simulink model "sistema"  (R2022b)
settings: Solver=ode4  StartTime=0.0  StopTime=4  FixedStep=1e-2  RelTol=1e-3  EnableMultiTasking=on
undefined symbols (not defined in the file): a, B, ft, K, l0, Lprime, M, R
settings Model: Creator=11802972  LastModifiedBy=andre
settings SolverCC: AlgebraicLoopSolver=TrustRegion
settings DataIOCC: LimitDataPoints=on  SaveFormat=Array  ReturnWorkspaceOutputs=off
settings OptimizationCC: LifeSpan=inf
settings DebuggingCC: UnconnectedInputMsg=warning  UnconnectedOutputMsg=warning  UnconnectedLineMsg=warning  SFUnexpectedBacktrackingDiag=warning  SFNoUnconditionalDefaultTransitionDiag=warning  SFExecutionAtInitializationDiag=none  SFMachineParentedDataDiag=warning  ArithmeticOperatorsInVariantConditions=warning
settings HardwareCC: ProdBitPerPointer=32  ProdBitPerSizeT=32  ProdBitPerPtrDiffT=32  ProdLargestAtomicFloat=None  ProdIntDivRoundTo=Undefined  ProdEndianess=Unspecified  ProdWordSize=32  ProdHWDeviceType=32-bit Generic
settings ModelReferenceCC: PropagateSignalLabelsOutOfModel=off
settings SFSimCC: SimUseLocalCustomCode=off  CustomCodeUndefinedFunction=UseInterfaceOnly
settings RTWCC: RTWUseLocalCustomCode=off
settings CodeAppCC: StateflowObjectComments=on
settings GRTTargetCC: TargetLangStandard=C89/C90 (ANSI)
settings ConfigComp: CovMetricSettings=dw  CovSaveCumulativeToWorkspaceVar=on  CovSaveSingleToWorkspaceVar=on  CovExternalEMLEnable=off

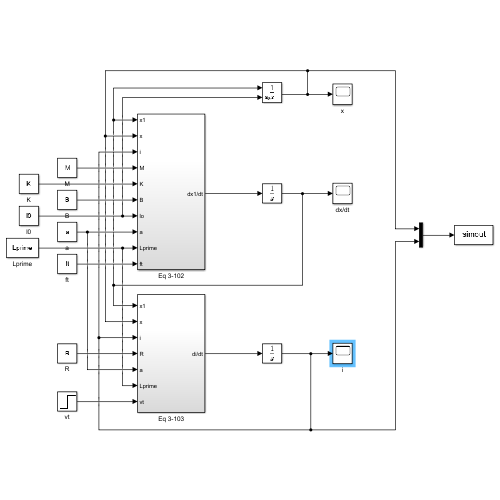
[thumbnail: Simulink's stored preview of the top-level diagram]
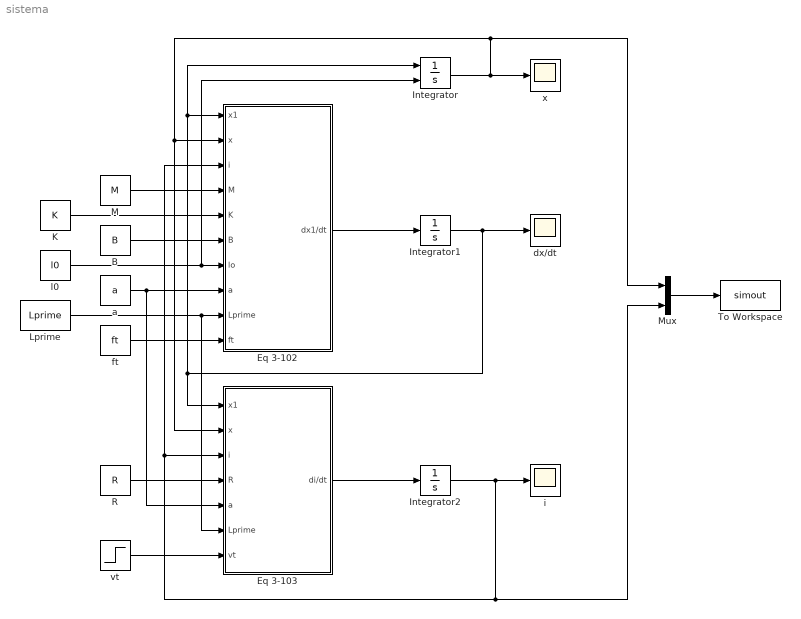
== system sistema ==
  B : Constant  Value=B
  "Eq 3-102 " : Subsystem
  Eq 3-103 : Subsystem
  Integrator : Integrator  InitialConditionSource=external
  Integrator1 : Integrator
  Integrator2 : Integrator
  K : Constant  Value=K
  Lprime : Constant  Value=Lprime
  M : Constant  Value=M
  Mux : Mux  Inputs=2
  R : Constant  Value=R
  To Workspace : ToWorkspace  VariableName=simout  SaveFormat=Timeseries  SampleTime=-1
  a : Constant  Value=a
  dx/dt : Scope
  ft : Constant  Value=ft
  i : Scope
  l0 : Constant  Value=l0
  "vt " : Step  Time=0.5  After=10  SampleTime=0
  x : Scope
  wires:
  M/1 -> "Eq 3-102 "/4(M)
  K/1 -> "Eq 3-102 "/5(K)
  B/1 -> "Eq 3-102 "/6(B)
  l0/1 -> Integrator/2, "Eq 3-102 "/7(lo)
  a/1 -> Eq 3-103/5(a), "Eq 3-102 "/8(a)
  ft/1 -> "Eq 3-102 "/10(ft)
  Lprime/1 -> Eq 3-103/6(Lprime), "Eq 3-102 "/9(Lprime)
  R/1 -> Eq 3-103/4(R)
  "vt "/1 -> Eq 3-103/7(vt)
  Integrator/1 -> Eq 3-103/2(x), "Eq 3-102 "/2(x), Mux/1, x/1
  "Eq 3-102 "/1(dx1/dt) -> Integrator1/1
  Integrator1/1 -> Eq 3-103/1(x1), Integrator/1, "Eq 3-102 "/1(x1), dx/dt/1
  Eq 3-103/1(di/dt) -> Integrator2/1
  Integrator2/1 -> Eq 3-103/3(i), "Eq 3-102 "/3(i), Mux/2, i/1
  Mux/1 -> To Workspace/1

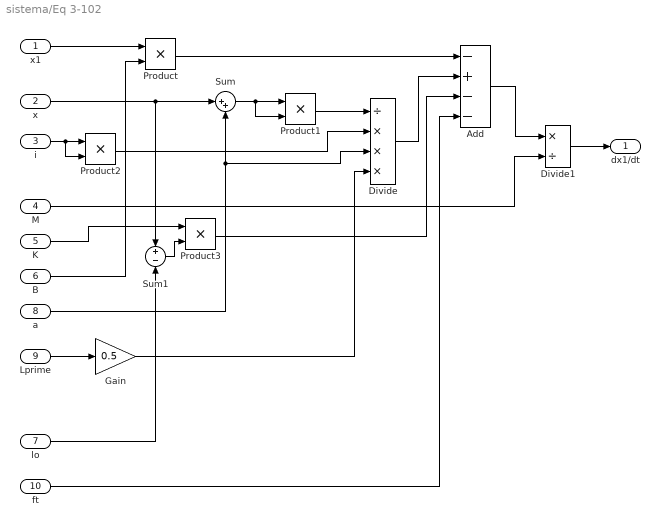
== system sistema/Eq 3-102  ==
  x1 : Inport
  x : Inport  Port=2
  i : Inport  Port=3
  M : Inport  Port=4
  K : Inport  Port=5
  B : Inport  Port=6
  lo : Inport  Port=7
  a : Inport  Port=8
  Lprime : Inport  Port=9
  ft : Inport  Port=10
  Add : Sum  Inputs=-+--
  Divide : Product  Inputs=/***
  Divide1 : Product  Inputs=*/
  Gain : Gain  Gain=0.5
  Product{,1..3} (4 alike) : Product
  Sum : Sum  Inputs=|++
  Sum1 : Sum  Inputs=+-
  dx1/dt : Outport
  wires:
  x1/1 -> Product/1
  B/1 -> Product/2
  Product/1 -> Add/1
  x/1 -> Sum/1, Sum1/1
  Sum/1 -> Product1/2, Product1/1
  a/1 -> Divide/3, Sum/2
  i/1 -> Product2/2, Product2/1
  Product1/1 -> Divide/1
  Product2/1 -> Divide/2
  Divide/1 -> Add/2
  Lprime/1 -> Gain/1
  Gain/1 -> Divide/4
  Sum1/1 -> Product3/2
  K/1 -> Product3/1
  lo/1 -> Sum1/2
  ft/1 -> Add/4
  Product3/1 -> Add/3
  Add/1 -> Divide1/1
  M/1 -> Divide1/2
  Divide1/1 -> dx1/dt/1

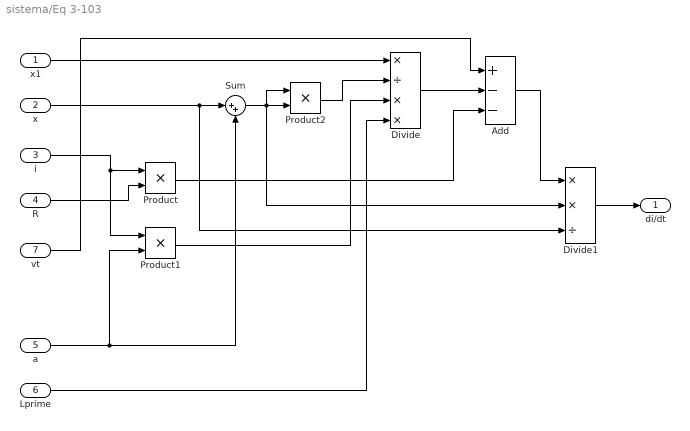
== system sistema/Eq 3-103 ==
  x1 : Inport
  x : Inport  Port=2
  i : Inport  Port=3
  R : Inport  Port=4
  a : Inport  Port=5
  Lprime : Inport  Port=6
  vt : Inport  Port=7
  Add : Sum  Inputs=+--
  Divide : Product  Inputs=*/**
  Divide1 : Product  Inputs=**/
  Product : Product
  Product1 : Product
  Product2 : Product
  Sum : Sum  Inputs=|++
  di/dt : Outport
  wires:
  i/1 -> Product1/1, Product/1
  R/1 -> Product/2
  a/1 -> Sum/2, Product1/2
  x/1 -> Divide1/3, Sum/1
  Sum/1 -> Divide1/2, Product2/1, Product2/2
  x1/1 -> Divide/1
  Product2/1 -> Divide/2
  Product1/1 -> Divide/3
  Lprime/1 -> Divide/4
  Divide/1 -> Add/2
  Product/1 -> Add/3
  vt/1 -> Add/1
  Add/1 -> Divide1/1
  Divide1/1 -> di/dt/1
